simulink model "SS6_Estimation"  (R2014b)
settings: Solver=ode45  StartTime=0.0  StopTime=50.0  RelTol=1e-3
settings Model: Creator=Bismaya  LastModifiedBy=Bismaya

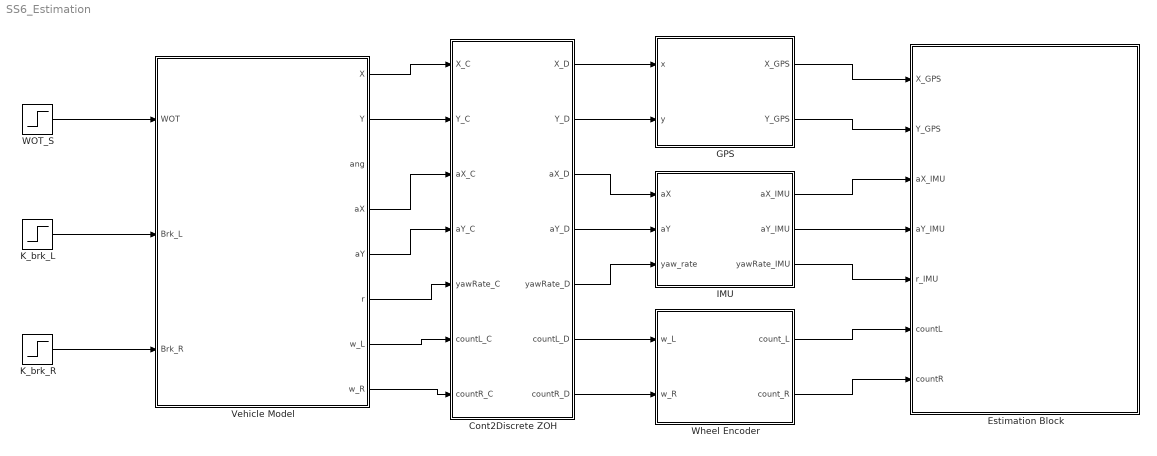
== system SS6_Estimation ==
  Cont2Discrete ZOH : Subsystem
  Estimation Block : Subsystem
  GPS : MATLAB Function  TreatAsAtomicUnit=on
  IMU : MATLAB Function  TreatAsAtomicUnit=on
  K_brk_L : Step  Time=0  After=0  SampleTime=0
  K_brk_R : Step  Time=20  SampleTime=0
  Vehicle Model : Subsystem
  "WOT_S " : Step  Time=0  Before=1  SampleTime=0
  Wheel Encoder : MATLAB Function  TreatAsAtomicUnit=on
  wires:
  "WOT_S "/1 -> Vehicle Model/1(WOT)
  K_brk_L/1 -> Vehicle Model/2(Brk_L)
  K_brk_R/1 -> Vehicle Model/3(Brk_R)
  Vehicle Model/1(X) -> Cont2Discrete ZOH/1(X_C)
  Vehicle Model/2(Y) -> Cont2Discrete ZOH/2(Y_C)
  Vehicle Model/4(aX) -> Cont2Discrete ZOH/3(aX_C)
  Vehicle Model/5(aY) -> Cont2Discrete ZOH/4(aY_C)
  Vehicle Model/6(r) -> Cont2Discrete ZOH/5(yawRate_C)
  Vehicle Model/7(w_L) -> Cont2Discrete ZOH/6(countL_C)
  Cont2Discrete ZOH/1(X_D) -> GPS/1(x)
  Cont2Discrete ZOH/2(Y_D) -> GPS/2(y)
  Cont2Discrete ZOH/3(aX_D) -> IMU/1(aX)
  Cont2Discrete ZOH/4(aY_D) -> IMU/2(aY)
  Cont2Discrete ZOH/5(yawRate_D) -> IMU/3(yaw_rate)
  Cont2Discrete ZOH/6(countL_D) -> Wheel Encoder/1(w_L)
  Cont2Discrete ZOH/7(countR_D) -> Wheel Encoder/2(w_R)
  GPS/1(X_GPS) -> Estimation Block/1(X_GPS)
  GPS/2(Y_GPS) -> Estimation Block/2(Y_GPS)
  IMU/1(aX_IMU) -> Estimation Block/3(aX_IMU)
  IMU/2(aY_IMU) -> Estimation Block/4(aY_IMU)
  IMU/3(yawRate_IMU) -> Estimation Block/5(r_IMU)
  Wheel Encoder/1(count_L) -> Estimation Block/6(countL)
  Wheel Encoder/2(count_R) -> Estimation Block/7(countR)
  Vehicle Model/8(w_R) -> Cont2Discrete ZOH/7(countR_C)

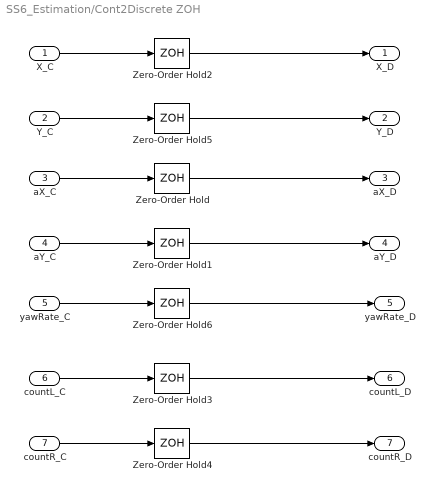
== system SS6_Estimation/Cont2Discrete ZOH ==
  X_C : Inport
  Y_C : Inport  Port=2
  aX_C : Inport  Port=3
  aY_C : Inport  Port=4
  yawRate_C : Inport  Port=5
  countL_C : Inport  Port=6
  countR_C : Inport  Port=7
  Zero-Order Hold{,1..6} (7 alike) : ZeroOrderHold  SampleTime=0.01
  X_D : Outport
  Y_D : Outport  Port=2
  aX_D : Outport  Port=3
  aY_D : Outport  Port=4
  yawRate_D : Outport  Port=5
  countL_D : Outport  Port=6
  countR_D : Outport  Port=7
  wires:
  Zero-Order Hold5/1 -> Y_D/1
  Zero-Order Hold2/1 -> X_D/1
  yawRate_C/1 -> Zero-Order Hold6/1
  aX_C/1 -> Zero-Order Hold/1
  aY_C/1 -> Zero-Order Hold1/1
  Y_C/1 -> Zero-Order Hold5/1
  X_C/1 -> Zero-Order Hold2/1
  countR_C/1 -> Zero-Order Hold4/1
  countL_C/1 -> Zero-Order Hold3/1
  Zero-Order Hold/1 -> aX_D/1
  Zero-Order Hold4/1 -> countR_D/1
  Zero-Order Hold3/1 -> countL_D/1
  Zero-Order Hold6/1 -> yawRate_D/1
  Zero-Order Hold1/1 -> aY_D/1

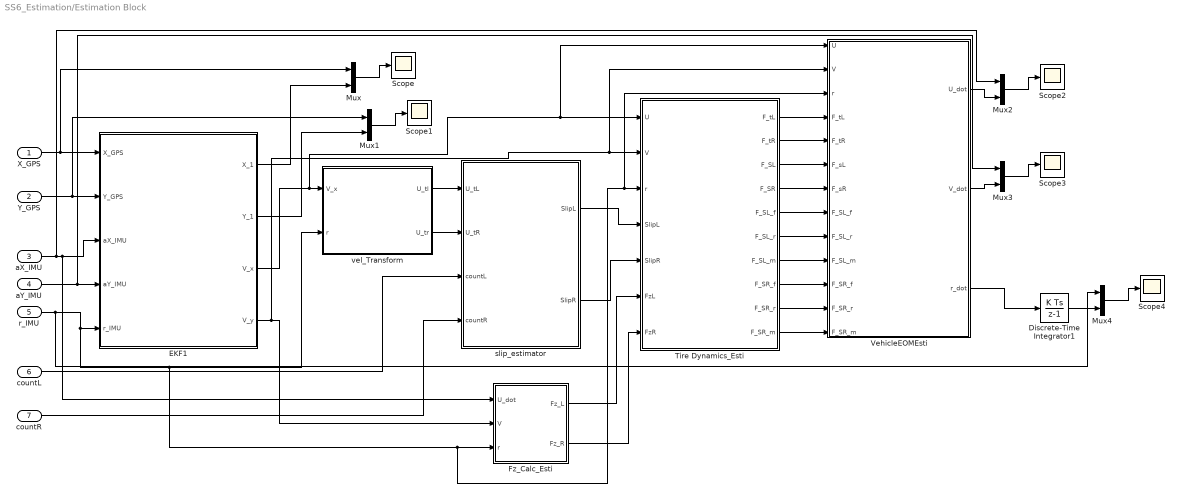
== system SS6_Estimation/Estimation Block ==
  X_GPS : Inport
  Y_GPS : Inport  Port=2
  aX_IMU : Inport  Port=3
  aY_IMU : Inport  Port=4
  r_IMU : Inport  Port=5
  countL : Inport  Port=6
  countR : Inport  Port=7
  Discrete-Time Integrator1 : DiscreteIntegrator  InitialConditionSetting=State (most efficient)  SampleTime=-1
  EKF1 : MATLAB Function  TreatAsAtomicUnit=on
  Fz_Calc_Esti : MATLAB Function  TreatAsAtomicUnit=on
  Mux{,1..4} (5 alike) : Mux  Inputs=2
  Scope{,1..4} (5 alike) : Scope
      Scope settings: SaveName=X_Comp
      Scope1 settings: SaveName=YComp
      Scope2 settings: SaveName=X_Comp1
      Scope3 settings: SaveName=X_Comp2
      Scope4 settings: SaveName=X_Comp3
  Tire Dynamics_Esti : Subsystem
  VehicleEOMEsti : MATLAB Function  TreatAsAtomicUnit=on
  slip_estimator : MATLAB Function  TreatAsAtomicUnit=on
  vel_Transform : MATLAB Function  TreatAsAtomicUnit=on
  wires:
  slip_estimator/1(SlipL) -> Tire Dynamics_Esti/4(SlipL)
  Tire Dynamics_Esti/10(F_SR_m) -> VehicleEOMEsti/13(F_SR_m)
  slip_estimator/2(SlipR) -> Tire Dynamics_Esti/5(SlipR)
  X_GPS/1 -> Mux/1, EKF1/1(X_GPS)
  aY_IMU/1 -> Mux3/1, EKF1/4(aY_IMU)
  aX_IMU/1 -> Mux2/1, Fz_Calc_Esti/1(U_dot), EKF1/3(aX_IMU)
  vel_Transform/2(U_tr) -> slip_estimator/2(U_tR)
  vel_Transform/1(U_tl) -> slip_estimator/1(U_tL)
  Fz_Calc_Esti/2(Fz_R) -> Tire Dynamics_Esti/7(FzR)
  Tire Dynamics_Esti/7(F_SL_m) -> VehicleEOMEsti/10(F_SL_m)
  Tire Dynamics_Esti/6(F_SL_r) -> VehicleEOMEsti/9(F_SL_r)
  Tire Dynamics_Esti/9(F_SR_r) -> VehicleEOMEsti/12(F_SR_r)
  Tire Dynamics_Esti/8(F_SR_f) -> VehicleEOMEsti/11(F_SR_f)
  Tire Dynamics_Esti/5(F_SL_f) -> VehicleEOMEsti/8(F_SL_f)
  Fz_Calc_Esti/1(Fz_L) -> Tire Dynamics_Esti/6(FzL)
  Tire Dynamics_Esti/1(F_tL) -> VehicleEOMEsti/4(F_tL)
  Tire Dynamics_Esti/3(F_SL) -> VehicleEOMEsti/6(F_sL)
  Tire Dynamics_Esti/2(F_tR) -> VehicleEOMEsti/5(F_tR)
  Tire Dynamics_Esti/4(F_SR) -> VehicleEOMEsti/7(F_sR)
  Mux/1 -> Scope/1
  EKF1/1(X_1) -> Mux/2
  Y_GPS/1 -> Mux1/1, EKF1/2(Y_GPS)
  Mux1/1 -> Scope1/1
  EKF1/2(Y_1) -> Mux1/2
  countL/1 -> slip_estimator/3(countL)
  countR/1 -> slip_estimator/4(countR)
  EKF1/3(V_x) -> VehicleEOMEsti/1(U), Tire Dynamics_Esti/1(U), vel_Transform/1(V_x)
  EKF1/4(V_y) -> VehicleEOMEsti/2(V), Tire Dynamics_Esti/2(V), Fz_Calc_Esti/2(V)
  r_IMU/1 -> Mux4/1, VehicleEOMEsti/3(r), Tire Dynamics_Esti/3(r), Fz_Calc_Esti/3(r), vel_Transform/2(r), EKF1/5(r_IMU)
  Mux2/1 -> Scope2/1
  VehicleEOMEsti/1(U_dot) -> Mux2/2
  Mux3/1 -> Scope3/1
  VehicleEOMEsti/2(V_dot) -> Mux3/2
  Mux4/1 -> Scope4/1
  Discrete-Time Integrator1/1 -> Mux4/2
  VehicleEOMEsti/3(r_dot) -> Discrete-Time Integrator1/1

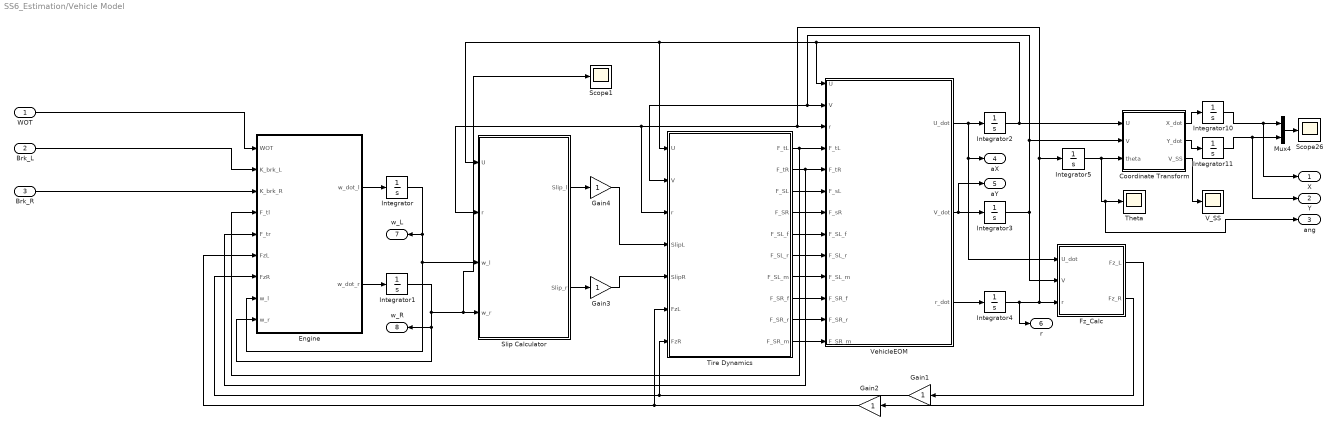
== system SS6_Estimation/Vehicle Model ==
  WOT : Inport
  Brk_L : Inport  Port=2
  Brk_R : Inport  Port=3
  Coordinate Transform : MATLAB Function  TreatAsAtomicUnit=on
  Engine : MATLAB Function  TreatAsAtomicUnit=on
  Fz_Calc : MATLAB Function  TreatAsAtomicUnit=on
  Gain{1..4} (4 alike) : Gain
  Integrator : Integrator  InitialCondition=12  LowerSaturationLimit=-0.0001
  Integrator1 : Integrator  InitialCondition=12  LowerSaturationLimit=-0.0001
  Integrator{3..5,10..11} (5 alike) : Integrator
  Integrator2 : Integrator  InitialCondition=10/3
  Mux4 : Mux  Inputs=2
  Scope1 : Scope
      settings: YMin=-50  YMax=200  SaveName=XY1
  Scope26 : Scope
      settings: YMin=-50  YMax=200  SaveName=XY
  Slip Calculator : MATLAB Function  TreatAsAtomicUnit=on
  Theta : Scope
      settings: YMin=20  YMax=45  SaveName=Theta
  Tire Dynamics : Subsystem
  V_SS : Scope
      settings: YMin=20  YMax=45  SaveName=Theta1
  VehicleEOM : MATLAB Function  TreatAsAtomicUnit=on
  X : Outport
  Y : Outport  Port=2
  ang : Outport  Port=3
  aX : Outport  Port=4
  aY : Outport  Port=5
  r : Outport  Port=6
  w_L : Outport  Port=7
  w_R : Outport  Port=8
  wires:
  Engine/1(w_dot_l) -> Integrator/1
  Integrator1/1 -> w_R/1, Engine/9(w_r), Scope1/1, Slip Calculator/4(w_r)
  Tire Dynamics/9(F_SR_r) -> VehicleEOM/12(F_SR_r)
  Tire Dynamics/8(F_SR_f) -> VehicleEOM/11(F_SR_f)
  Tire Dynamics/5(F_SL_f) -> VehicleEOM/8(F_SL_f)
  Tire Dynamics/7(F_SL_m) -> VehicleEOM/10(F_SL_m)
  Brk_L/1 -> Engine/2(K_brk_L)
  Integrator/1 -> w_L/1, Slip Calculator/3(w_l), Engine/8(w_l)
  Brk_R/1 -> Engine/3(K_brk_R)
  Tire Dynamics/1(F_tL) -> Engine/4(F_tl), VehicleEOM/4(F_tL)
  Engine/2(w_dot_r) -> Integrator1/1
  Tire Dynamics/4(F_SR) -> VehicleEOM/7(F_sR)
  VehicleEOM/1(U_dot) -> aX/1, Fz_Calc/1(U_dot), Integrator2/1
  VehicleEOM/2(V_dot) -> aY/1, Integrator3/1
  VehicleEOM/3(r_dot) -> Integrator4/1
  Integrator2/1 -> Tire Dynamics/1(U), Slip Calculator/1(U), VehicleEOM/1(U), Coordinate Transform/1(U)
  Integrator3/1 -> Tire Dynamics/2(V), VehicleEOM/2(V), Coordinate Transform/2(V), Fz_Calc/2(V)
  Fz_Calc/2(Fz_R) -> Gain1/1
  Fz_Calc/1(Fz_L) -> Gain2/1
  Slip Calculator/2(Slip_r) -> Gain3/1
  Tire Dynamics/2(F_tR) -> Engine/5(F_tr), VehicleEOM/5(F_tR)
  Integrator4/1 -> r/1, Tire Dynamics/3(r), Slip Calculator/2(r), VehicleEOM/3(r), Integrator5/1, Fz_Calc/3(r)
  Integrator5/1 -> Coordinate Transform/3(theta), ang/1, Theta/1
  Coordinate Transform/1(X_dot) -> Integrator10/1
  Slip Calculator/1(Slip_l) -> Gain4/1
  WOT/1 -> Engine/1(WOT)
  Tire Dynamics/10(F_SR_m) -> VehicleEOM/13(F_SR_m)
  Tire Dynamics/6(F_SL_r) -> VehicleEOM/9(F_SL_r)
  Tire Dynamics/3(F_SL) -> VehicleEOM/6(F_sL)
  Gain1/1 -> Engine/7(FzR), Tire Dynamics/7(FzR)
  Gain3/1 -> Tire Dynamics/5(SlipR)
  Gain2/1 -> Engine/6(FzL), Tire Dynamics/6(FzL)
  Gain4/1 -> Tire Dynamics/4(SlipL)
  Coordinate Transform/2(Y_dot) -> Integrator11/1
  Integrator10/1 -> X/1, Mux4/1
  Integrator11/1 -> Y/1, Mux4/2
  Mux4/1 -> Scope26/1
  Coordinate Transform/3(V_SS) -> V_SS/1

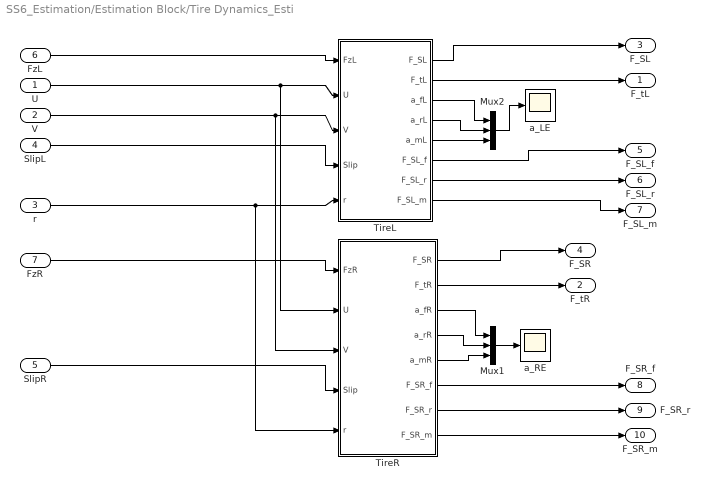
== system SS6_Estimation/Estimation Block/Tire Dynamics_Esti ==
  U : Inport
  V : Inport  Port=2
  r : Inport  Port=3
  SlipL : Inport  Port=4
  SlipR : Inport  Port=5
  FzL : Inport  Port=6
  FzR : Inport  Port=7
  Mux1 : Mux  Inputs=3
  Mux2 : Mux  Inputs=3
  TireL : MATLAB Function  TreatAsAtomicUnit=on
  TireR : MATLAB Function  TreatAsAtomicUnit=on
  a_LE : Scope
      settings: YMin=20  YMax=45  SaveName=a_LE  MaxDataPoints=5000000
  a_RE : Scope
      settings: YMin=20  YMax=45  SaveName=a_RE  MaxDataPoints=5000000
  F_tL : Outport
  F_tR : Outport  Port=2
  F_SL : Outport  Port=3
  F_SR : Outport  Port=4
  F_SL_f : Outport  Port=5
  F_SL_r : Outport  Port=6
  F_SL_m : Outport  Port=7
  F_SR_f : Outport  Port=8
  F_SR_r : Outport  Port=9
  F_SR_m : Outport  Port=10
  wires:
  TireL/8(F_SL_m) -> F_SL_m/1
  U/1 -> TireL/2(U), TireR/2(U)
  FzR/1 -> TireR/1(FzR)
  SlipR/1 -> TireR/4(Slip)
  V/1 -> TireR/3(V), TireL/3(V)
  TireR/1(F_SR) -> F_SR/1
  r/1 -> TireR/5(r), TireL/5(r)
  TireL/2(F_tL) -> F_tL/1
  TireL/6(F_SL_f) -> F_SL_f/1
  SlipL/1 -> TireL/4(Slip)
  TireL/7(F_SL_r) -> F_SL_r/1
  FzL/1 -> TireL/1(FzL)
  TireL/1(F_SL) -> F_SL/1
  Mux2/1 -> a_LE/1
  TireR/3(a_fR) -> Mux1/1
  TireR/4(a_rR) -> Mux1/2
  Mux1/1 -> a_RE/1
  TireR/5(a_mR) -> Mux1/3
  TireR/2(F_tR) -> F_tR/1
  TireR/6(F_SR_f) -> F_SR_f/1
  TireR/7(F_SR_r) -> F_SR_r/1
  TireR/8(F_SR_m) -> F_SR_m/1
  TireL/5(a_mL) -> Mux2/3
  TireL/3(a_fL) -> Mux2/1
  TireL/4(a_rL) -> Mux2/2

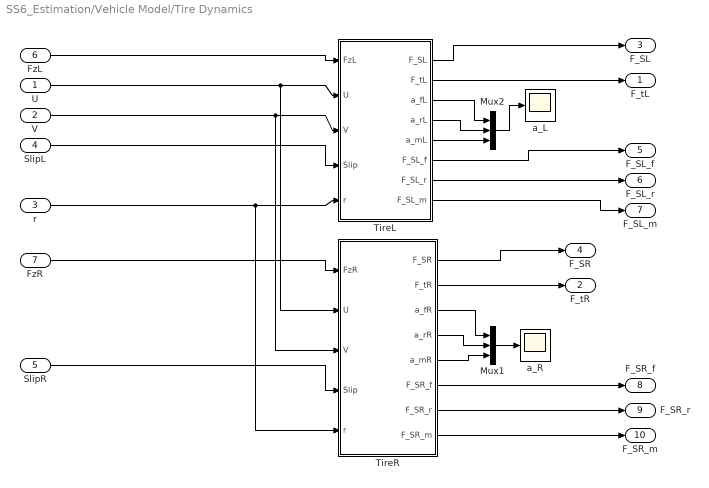
== system SS6_Estimation/Vehicle Model/Tire Dynamics ==
  U : Inport
  V : Inport  Port=2
  r : Inport  Port=3
  SlipL : Inport  Port=4
  SlipR : Inport  Port=5
  FzL : Inport  Port=6
  FzR : Inport  Port=7
  Mux1 : Mux  Inputs=3
  Mux2 : Mux  Inputs=3
  TireL : MATLAB Function  TreatAsAtomicUnit=on
  TireR : MATLAB Function  TreatAsAtomicUnit=on
  a_L : Scope
      settings: YMin=20  YMax=45  SaveName=a_L  MaxDataPoints=5000000
  a_R : Scope
      settings: YMin=20  YMax=45  SaveName=a_R  MaxDataPoints=5000000
  F_tL : Outport
  F_tR : Outport  Port=2
  F_SL : Outport  Port=3
  F_SR : Outport  Port=4
  F_SL_f : Outport  Port=5
  F_SL_r : Outport  Port=6
  F_SL_m : Outport  Port=7
  F_SR_f : Outport  Port=8
  F_SR_r : Outport  Port=9
  F_SR_m : Outport  Port=10
  wires:
  TireL/8(F_SL_m) -> F_SL_m/1
  U/1 -> TireL/2(U), TireR/2(U)
  FzR/1 -> TireR/1(FzR)
  SlipR/1 -> TireR/4(Slip)
  V/1 -> TireR/3(V), TireL/3(V)
  TireR/1(F_SR) -> F_SR/1
  r/1 -> TireR/5(r), TireL/5(r)
  TireL/2(F_tL) -> F_tL/1
  TireL/6(F_SL_f) -> F_SL_f/1
  SlipL/1 -> TireL/4(Slip)
  TireL/7(F_SL_r) -> F_SL_r/1
  FzL/1 -> TireL/1(FzL)
  TireL/1(F_SL) -> F_SL/1
  Mux2/1 -> a_L/1
  TireR/3(a_fR) -> Mux1/1
  TireR/4(a_rR) -> Mux1/2
  Mux1/1 -> a_R/1
  TireR/5(a_mR) -> Mux1/3
  TireR/2(F_tR) -> F_tR/1
  TireR/6(F_SR_f) -> F_SR_f/1
  TireR/7(F_SR_r) -> F_SR_r/1
  TireR/8(F_SR_m) -> F_SR_m/1
  TireL/5(a_mL) -> Mux2/3
  TireL/3(a_fL) -> Mux2/1
  TireL/4(a_rL) -> Mux2/2

== matlab function SS6_Estimation/GPS ==
  data: x input; y input; X_GPS output; Y_GPS output
function [X_GPS,Y_GPS] = GPS_fcn(x,y)
%#codegen

X_GPS=x+0.0001*randn(1);
Y_GPS=y+0.0001*randn(1);

== matlab function SS6_Estimation/Vehicle Model/Engine ==
  data: WOT input; K_brk_L input; K_brk_R input; F_tl input; F_tr input; FzL input; FzR input; w_l input; w_r input; w_dot_l output; w_dot_r output
function [w_dot_l,w_dot_r] = engine_model(WOT,K_brk_L,K_brk_R,F_tl,F_tr,FzL,FzR,w_l,w_r)
M=1280;Ms=1160;Izz=2500;Ixx=750;Ixz=0;a=1.203;b=1.217;hcg=0.5;e=0.2;Tw=1.33;R=0.3;I_t=2.1;
I_e=0.136;A_f=2.1;zi1=2.5*13.56;zi2=7.50;zi3=5.37;zi4=4.22;zi5=3.28;
Lbpsi=45000;Lbp=2600;C_a=20000;C_i=20000;mu=0.85;e_r=0.015;K_rsf=-0.05;K_rsr=0.1;
C1=-6.0;C2=59.16;C3=25;C_s1=1.38;K_rsf=0.444;C_d=0.32;d=0.014;n=0.85;
rho=1.204;g=9.81;
K_bf=0.55;
zi=zi1*2;

F_tl=F_tl;
F_tr=F_tr;
F_t1=F_tl+F_tr;
%Engine Equations
w_el=zi*w_l;
w_er=zi*w_r;

IwL=I_t+(0.5*zi*zi*n*I_e);%Accelerating
IwR=I_t+(0.5*zi*zi*n*I_e);%Accelerating

T_l=WOT*zi*n*(C1*(w_el/100)^2+C2*(w_el/100)+C3);
T_r=WOT*zi*n*(C1*(w_er/100)^2+C2*(w_er/100)+C3);
T_trac_L=T_l-(R*F_tl)-(d*FzL);
T_trac_R=T_r-(R*F_tr)-(d*FzR);
T_brkl=K_brk_L*T_l;
T_brkr=K_brk_R*T_r;
w_dot_l=(1/(IwL))*(T_trac_L-T_brkl);
w_dot_r=(1/(IwR))*(T_trac_R-T_brkr);
% w_dot_f=(1/Iw)*(T_f-(d*Fzf)-(0.5*T_brkf));
% w_dot_r=(1/Iw)*(T_r-(d*Fzr)-(0.5*T_brkr));

== matlab function SS6_Estimation/Vehicle Model/Tire Dynamics/TireR ==
  data: FzR input; F_SR output; F_tR output; U input; V input; Slip input; r input; a_fR output; a_rR output; a_mR output; F_SR_f output; F_SR_r output; F_SR_m output
function [F_SR,F_tR,a_fR,a_rR,a_mR,F_SR_f,F_SR_r,F_SR_m] = tireR(FzR,U,V,Slip,r)
M=1280;Ms=1160;Izz=2500;Ixx=750;Ixz=0;a=1.203;b=1.217;hcg=0.5;e=0.2;Tw=1.33;R=0.3;I_t=2.1;
I_e=0.136;A_f=2.1;K_bf=0.55;zi1=13.56;z2=7.50;zi3=5.37;zi4=4.22;zi5=3.28;
Lbpsi=45000;Lbp=2600;C_a=20000;C_i=20000;mu=0.85;e_r=0.015;K_rsf=-0.05;K_rsr=0.1;
C1=-6.0;C2=59.16;C3=25;C_s1=1.38;K_rsf=0.444;C_d=0.32;d=0.014;n=0.85;
rho=1.204;g=9.81;c=0.2;


% FzF=M*g*mu/2;
Fz=FzR;

%Tire Longitudinal Velocity Calculation
% U_tf=U*cos(delta)+(V+a*r)*sin(delta);
% U_tr=U;

 %Side Slip Calc
a_fR=-atan((V+a*r)/(U-0.5*Tw*r));
a_rR=atan((b*r-V)/(U-0.5*Tw*r));
a_mR=atan((c*r-V)/(U-0.5*Tw*r));

alpha=a_fR;

 U_tl=U+(0.5*Tw*r);
 U_tr=U-(0.5*Tw*r);
%%FRONT Tires
%Tire Equations
S_f=(mu*(Fz/3)*(1-(e_r*U_tr*sqrt((Slip*Slip)+(tan(alpha)*tan(alpha)))))*(1-Slip))/...
    (2*sqrt(C_i*C_i*Slip*Slip+C_a*C_a*tan(alpha)*tan(alpha)));
if(S_f<1)
    f_S=S_f*(2-S_f);
else
    f_S=1;
end
F_SR_f=(C_a*tan(alpha)*f_S)/(1-Slip);
F_tR_f=(C_i*Slip*f_S)/(1-Slip);

%%Rear Tires
alpha=a_rR;

S_r=(mu*(Fz/3)*(1-(e_r*U_tr*sqrt((Slip*Slip)+(tan(alpha)*tan(alpha)))))*(1-Slip))/...
    (2*sqrt(C_i*C_i*Slip*Slip+C_a*C_a*tan(alpha)*tan(alpha)));
if(S_r<1)
    f_S=S_r*(2-S_r);
else
    f_S=1;
end
F_SR_r=(C_a*tan(alpha)*f_S)/(1-Slip);
F_tR_r=(C_i*Slip*f_S)/(1-Slip);

%%Middle Tires
alpha=a_mR;

S_m=(mu*(Fz/3)*(1-(e_r*U_tr*sqrt((Slip*Slip)+(tan(alpha)*tan(alpha)))))*(1-Slip))/...
    (2*sqrt(C_i*C_i*Slip*Slip+C_a*C_a*tan(alpha)*tan(alpha)));
if(S_m<1)
    f_S=S_m*(2-S_m);
else
    f_S=1;
end
F_SR_m=(C_a*tan(alpha)*f_S)/(1-Slip);
F_tR_m=(C_i*Slip*f_S)/(1-Slip);


F_SR=F_SR_f+F_SR_r+F_SR_m;
F_tR=F_tR_f+F_tR_r+F_tR_m;
F_R=[F_tR_f;F_tR_r;F_tR_m;F_SR_f;F_SR_r;F_SR_m];

== matlab function SS6_Estimation/Vehicle Model/VehicleEOM ==
  data: U input; V input; U_dot output; V_dot output; r input; F_tL input; F_tR input; F_sL input; F_sR input; r_dot output; F_SL_f input; F_SL_r input; F_SL_m input; F_SR_f input; F_SR_r input; F_SR_m input
function [U_dot,V_dot,r_dot] = VehicleEOM(U,V,r,F_tL,F_tR,F_sL,F_sR,F_SL_f,F_SL_r,F_SL_m,F_SR_f,F_SR_r,F_SR_m)
M=1280;Ms=1160;Izz=2500;Ixx=750;Ixz=0;a=1.203;b=1.217;hcg=0.5;e=0.2;Tw=1.33;R=0.3;I_t=2.1;
I_e=0.136;A_f=2.1;K_bf=0.55;zi1=13.56;z2=7.50;zi3=5.37;zi4=4.22;zi5=3.28;
Lbpsi=45000;Lbp=2600;C_a=20000;C_i=20000;mu=0.85;e_r=0.015;K_rsf=-0.05;K_rsr=0.1;
C1=-6.0;C2=59.16;C3=25;C_s1=1.38;K_rsf=0.444;C_d=0.32;d=0.014;n=0.85;
rho=1.204;g=9.81;c=0.2;

F_t=(F_tL+F_tR);
%Vehicle Equations
% U_dot=(1/M)*((M*V*r)+F_t-(0.5*C_d*A_f*rho*U*U));
U_dot=(1/M)*((M*V*r)+F_t);

V_dot=(1/M)*((-M*U*r)+F_sL+F_sR);
% r_dot=(1/Izz)*(2*a*F_tL*sin(delta)+2*a*F_sL*cos(delta)-2*b*F_sR);
 r_dot=(1/(0.5*Izz))*(0.5*Tw*F_tL-0.5*Tw*F_tR+a*(F_SL_f+F_SR_f)-b*(F_SL_r+F_SR_r)-c*(F_SL_m+F_SR_m));

== matlab function SS6_Estimation/Vehicle Model/Slip Calculator ==
  data: U input; r input; w_l input; w_r input; Slip_l output; Slip_r output
function [Slip_l,Slip_r] = slipCalculator(U,r,w_l,w_r)
M=1280;Ms=1160;Izz=2500;Ixx=750;Ixz=0;a=1.203;b=1.217;hcg=0.5;e=0.2;Tw=1.33;R=0.3;I_t=2.1;
I_e=0.136;A_f=2.1;K_bf=0.55;zi1=13.56;z2=7.50;zi3=5.37;zi4=4.22;zi5=3.28;
Lbpsi=45000;Lbp=2600;C_a=20000;C_i=20000;mu=0.85;e_r=0.015;K_rsf=-0.05;K_rsr=0.1;
C1=-6.0;C2=59.16;C3=25;C_s1=1.38;K_rsf=0.444;C_d=0.32;d=0.014;n=0.85;
rho=1.204;g=9.81;

% w_r=-w_r;
% w_f=-w_f;
%Tire Longitudinal Velocity Calculation
% U_tl=U*cos(delta)+(V+a*r)*sin(delta);
% U_tr=U;
 U_tl=U+(0.5*Tw*r);
 U_tr=U-(0.5*Tw*r);

% %  SlipCalc
% if(U_tl<=(R*w_l))
%     Slip_l=1-(U_tl/(R*w_l));%Acceleration
% else
%     Slip_l=1-((R*w_l)/U_tl);%Braking
% %     Slip_l=0;
% end
% 
% if(U_tr<=(R*w_r))
%     Slip_r=1-(U_tr/(R*w_r));%Acceleration
% else
%     Slip_r=1-((R*w_r)/U_tr);%Braking
% %     Slip_r=0;
% end
Slip_l=1-(U_tl/(R*w_l));
Slip_r=1-(U_tr/(R*w_r));

% 
% if(Slip_l<0)
%      Slip_l=0;
%  elseif (Slip_l>1)
%          Slip_l=1;
%  end
%  if(Slip_r<0)
%      Slip_r=0;
%  elseif (Slip_r>1)
%          Slip_r=1;
%  end
% %

== matlab function SS6_Estimation/Vehicle Model/Fz_Calc ==
  data: U_dot input; V input; Fz_L output; Fz_R output; r input
function [Fz_L,Fz_R] = FzCalc(U_dot,V,r)
M=1280;Ms=1160;Izz=2500;Ixx=750;Ixz=0;a=1.203;b=1.217;hcg=0.5;e=0.2;Tw=1.33;R=0.3;I_t=2.1;
I_e=0.136;A_f=2.1;K_bf=0.55;zi1=13.56;z2=7.50;zi3=5.37;zi4=4.22;zi5=3.28;
Lbpsi=45000;Lbp=2600;C_a=20000;C_i=20000;mu=0.85;e_r=0.015;K_rsf=-0.05;K_rsr=0.1;
C1=-6.0;C2=59.16;C3=25;C_s1=1.38;K_rsf=0.444;C_d=0.32;d=0.014;n=0.85;
rho=1.204;g=9.81;


%NormalForceCalc
% Fz_f=(M*g/2)*((b/(a+b))-((U_dot-V*r)*hcg)/(g*(a+b)));
% Fz_r=(M*g/2)*((a/(a+b))+((U_dot-V*r)*hcg)/(g*(a+b)));
Fz_L=(M*g/2);
Fz_R=(M*g/2);

== matlab function SS6_Estimation/Vehicle Model/Tire Dynamics/TireL ==
  data: FzL input; F_SL output; F_tL output; U input; V input; Slip input; r input; a_fL output; a_rL output; a_mL output; F_SL_f output; F_SL_r output; F_SL_m output
function [F_SL,F_tL,a_fL,a_rL,a_mL,F_SL_f,F_SL_r,F_SL_m] = tireL(FzL,U,V,Slip,r)
M=1280;Ms=1160;Izz=2500;Ixx=750;Ixz=0;a=1.203;b=1.217;hcg=0.5;e=0.2;Tw=1.33;R=0.3;I_t=2.1;
I_e=0.136;A_f=2.1;K_bf=0.55;zi1=13.56;z2=7.50;zi3=5.37;zi4=4.22;zi5=3.28;
Lbpsi=45000;Lbp=2600;C_a=20000;C_i=20000;mu=0.85;e_r=0.015;K_rsf=-0.05;K_rsr=0.1;
C1=-6.0;C2=59.16;C3=25;C_s1=1.38;K_rsf=0.444;C_d=0.32;d=0.014;n=0.85;
rho=1.204;g=9.81;c=0.2;


% FzF=M*g*mu/2;

Fz=FzL;

%Tire Longitudinal Velocity Calculation
% U_tf=U*cos(delta)+(V+a*r)*sin(delta);
% U_tr=U;
 U_tl=U+(0.5*Tw*r);
 U_tr=U-(0.5*Tw*r);
%FRONT Tires
 %Side Slip Calc
a_fL=-atan((V+a*r)/(U+0.5*Tw*r));
a_rL=atan((b*r-V)/(U+0.5*Tw*r));
a_mL=atan((c*r-V)/(U+0.5*Tw*r));

alpha=a_fL;
%Tire Equations
S_f=(mu*(Fz/3)*(1-(e_r*U_tl*sqrt((Slip*Slip)+(tan(alpha)*tan(alpha)))))*(1-Slip))/...
    (2*sqrt(C_i*C_i*Slip*Slip+C_a*C_a*tan(alpha)*tan(alpha)));
if(S_f<1)
    f_S=S_f*(2-S_f);
else
    f_S=1;
end
F_SL_f=(C_a*tan(alpha)*f_S)/(1-Slip);
F_tL_f=(C_i*Slip*f_S)/(1-Slip);

%Rear Tires
alpha=a_rL;

S_r=(mu*(Fz/3)*(1-(e_r*U_tl*sqrt((Slip*Slip)+(tan(alpha)*tan(alpha)))))*(1-Slip))/...
    (2*sqrt(C_i*C_i*Slip*Slip+C_a*C_a*tan(alpha)*tan(alpha)));
if(S_r<1)
    f_S=S_r*(2-S_r);
else
    f_S=1;
end
F_SL_r=(C_a*tan(alpha)*f_S)/(1-Slip);
F_tL_r=(C_i*Slip*f_S)/(1-Slip);

%Middle Tires
alpha=a_mL;

S_m=(mu*(Fz/3)*(1-(e_r*U_tl*sqrt((Slip*Slip)+(tan(alpha)*tan(alpha)))))*(1-Slip))/...
    (2*sqrt(C_i*C_i*Slip*Slip+C_a*C_a*tan(alpha)*tan(alpha)));
if(S_m<1)
    f_S=S_m*(2-S_m);
else
    f_S=1;
end
F_SL_m=(C_a*tan(alpha)*f_S)/(1-Slip);
F_tL_m=(C_i*Slip*f_S)/(1-Slip);


F_SL=F_SL_f+F_SL_r+F_SL_m;
F_tL=F_tL_f+F_tL_r+F_tL_m;
F_L=[F_tL_f;F_tL_r;F_tL_m;F_SL_f;F_SL_r;F_SL_m;];

== matlab function SS6_Estimation/Vehicle Model/Coordinate Transform ==
  data: U input; V input; theta input; X_dot output; Y_dot output; V_SS output
    function [X_dot,Y_dot, V_SS] = CT(U,V,theta)
M=1280;Ms=1160;Izz=2500;Ixx=750;Ixz=0;a=1.203;b=1.217;hcg=0.5;e=0.2;Tw=1.33;R=0.3;I_t=2.1;
I_e=0.136;A_f=2.1;K_bf=0.55;zi1=13.56;z2=7.50;zi3=5.37;zi4=4.22;zi5=3.28;
Lbpsi=45000;Lbp=2600;C_a=20000;C_i=20000;mu=0.85;e_r=0.015;K_rsf=-0.05;K_rsr=0.1;
C1=-6.0;C2=59.16;C3=25;C_s1=1.38;K_rsf=0.444;C_d=0.32;d=0.014;n=0.85;
rho=1.204;g=9.81;c=0.2;

X_dot=U*cos(theta)-V*sin(theta);
Y_dot=+U*sin(theta)+V*cos(theta);
% X_dot=U*sin(theta)+V*cos(theta);
% Y_dot=U*cos(theta)-V*sin(theta);
V_SS=atand(V/U);

== matlab function SS6_Estimation/IMU ==
  data: aX input; aY input; aX_IMU output; aY_IMU output; yaw_rate input; yawRate_IMU output
function [aX_IMU,aY_IMU,yawRate_IMU] = IMU_fcn(aX,aY,yaw_rate)
%#codegen

aX_IMU=aX+0.0001*randn(1);
aY_IMU=aY+0.0001*randn(1);
yawRate_IMU=yaw_rate+0.0001*randn(1);

== matlab function SS6_Estimation/Wheel Encoder ==
  data: w_L input; w_R input; count_L output; count_R output
function [count_L,count_R] = encoder_fcn(w_L,w_R)
%#codegen

count_L=w_L+0.0001*randn(1);
count_R=w_R+0.0001*randn(1);

== matlab function SS6_Estimation/Estimation Block/EKF1 ==
  data: X_1 output; Y_1 output; X_GPS input; Y_GPS input; aX_IMU input; aY_IMU input; r_IMU input; V_x output; V_y output
function [X_1,Y_1,V_x,V_y]  = EKF_fcn(X_GPS,Y_GPS,aX_IMU,aY_IMU,r_IMU)

persistent cov State 

if isempty(cov)
State=zeros(7,1);
cov=zeros(7);
end

% Motion Noise
Q=0.0001*eye(7);
Q(4:7,4:7)=0;
% Measurement Noise
R=0.0001*eye(2);
% Sampling Time
Ts=0.01;
% Control Matrix
B=[Ts 0 0;
    0 Ts 0;
    0 0 Ts;
    0 0 0;
    0 0 0;
    0 0 0;
    0 0 0;];

%Motion Jacobian
G=[ 1 0 0 0 0 0 0;
    0 1 0 0 0 0 0;
    0 0 1 0 0 0 0;
    cos(State(3)) -sin(State(3)) -State(1)*sin(State(3))-State(2)*cos(State(3)) 0 0 0 0;
    sin(State(3)) cos(State(3)) State(1)*cos(State(3))-State(2)*sin(State(3)) 0 0 0 0;
    0 0 0 Ts 0 1 0;
    0 0 0 0 Ts 0 1;];

% Motion Model 
g=[State(1);
    State(2);
    State(3);
    State(1)*cos(State(3))-State(2)*sin(State(3));
    State(1)*sin(State(3))+State(2)*cos(State(3));
    Ts*State(4)+State(6);
    Ts*State(5)+State(7);];

%Propagate the State and Covariance
State_p=g+B*[aX_IMU;
             aY_IMU;
             r_IMU;];
cov=G*cov*G'+Q;

H= [0 0 0 0 0 1 0;
    0 0 0 0 0 0 1;];
%     0 0 1 0 0 0 0;];
% Take Measurements
y_meas=[X_GPS;
        Y_GPS];
    
K=cov*H'*pinv(H*cov*H'+R);
State=State_p+K*(y_meas-H*State_p);
cov = (eye(7)-K*H)*cov;
X_1=State(6);
Y_1=State(7);
V_x=State(1);
V_y=State(2);
end

== matlab function SS6_Estimation/Estimation Block/vel_Transform ==
  data: V_x input; r input; U_tl output; U_tr output
function [U_tl,U_tr] = velocity_transform(V_x,r)
%#codegen
 Tw=1.33;
 U_tl=V_x+(0.5*Tw*r);
 U_tr=V_x-(0.5*Tw*r);
end

== matlab function SS6_Estimation/Estimation Block/slip_estimator ==
  data: U_tL input; U_tR input; SlipL output; SlipR output; countL input; countR input
function [SlipL,SlipR] = slip_estimator(U_tL,U_tR,countL,countR)
%#codegen
R=0.3;

SlipL=1-(U_tL/(R*countL));
SlipR=1-(U_tR/(R*countR));
end

== matlab function SS6_Estimation/Estimation Block/Tire Dynamics_Esti/TireL ==
  data: FzL input; F_SL output; F_tL output; U input; V input; Slip input; r input; a_fL output; a_rL output; a_mL output; F_SL_f output; F_SL_r output; F_SL_m output
function [F_SL,F_tL,a_fL,a_rL,a_mL,F_SL_f,F_SL_r,F_SL_m] = tireL(FzL,U,V,Slip,r)
M=1280;Ms=1160;Izz=2500;Ixx=750;Ixz=0;a=1.203;b=1.217;hcg=0.5;e=0.2;Tw=1.33;R=0.3;I_t=2.1;
I_e=0.136;A_f=2.1;K_bf=0.55;zi1=13.56;z2=7.50;zi3=5.37;zi4=4.22;zi5=3.28;
Lbpsi=45000;Lbp=2600;C_a=20000;C_i=20000;mu=0.85;e_r=0.015;K_rsf=-0.05;K_rsr=0.1;
C1=-6.0;C2=59.16;C3=25;C_s1=1.38;K_rsf=0.444;C_d=0.32;d=0.014;n=0.85;
rho=1.204;g=9.81;c=0.2;


% FzF=M*g*mu/2;

Fz=FzL;

%Tire Longitudinal Velocity Calculation
% U_tf=U*cos(delta)+(V+a*r)*sin(delta);
% U_tr=U;
 U_tl=U+(0.5*Tw*r);
 U_tr=U-(0.5*Tw*r);
%FRONT Tires
 %Side Slip Calc
a_fL=-atan((V+a*r)/(U+0.5*Tw*r));
a_rL=atan((b*r-V)/(U+0.5*Tw*r));
a_mL=atan((c*r-V)/(U+0.5*Tw*r));

alpha=a_fL;
%Tire Equations
S_f=(mu*(Fz/3)*(1-(e_r*U_tl*sqrt((Slip*Slip)+(tan(alpha)*tan(alpha)))))*(1-Slip))/...
    (2*sqrt(C_i*C_i*Slip*Slip+C_a*C_a*tan(alpha)*tan(alpha)));
if(S_f<1)
    f_S=S_f*(2-S_f);
else
    f_S=1;
end
F_SL_f=(C_a*tan(alpha)*f_S)/(1-Slip);
F_tL_f=(C_i*Slip*f_S)/(1-Slip);

%Rear Tires
alpha=a_rL;

S_r=(mu*(Fz/3)*(1-(e_r*U_tl*sqrt((Slip*Slip)+(tan(alpha)*tan(alpha)))))*(1-Slip))/...
    (2*sqrt(C_i*C_i*Slip*Slip+C_a*C_a*tan(alpha)*tan(alpha)));
if(S_r<1)
    f_S=S_r*(2-S_r);
else
    f_S=1;
end
F_SL_r=(C_a*tan(alpha)*f_S)/(1-Slip);
F_tL_r=(C_i*Slip*f_S)/(1-Slip);

%Middle Tires
alpha=a_mL;

S_m=(mu*(Fz/3)*(1-(e_r*U_tl*sqrt((Slip*Slip)+(tan(alpha)*tan(alpha)))))*(1-Slip))/...
    (2*sqrt(C_i*C_i*Slip*Slip+C_a*C_a*tan(alpha)*tan(alpha)));
if(S_m<1)
    f_S=S_m*(2-S_m);
else
    f_S=1;
end
F_SL_m=(C_a*tan(alpha)*f_S)/(1-Slip);
F_tL_m=(C_i*Slip*f_S)/(1-Slip);


F_SL=F_SL_f+F_SL_r+F_SL_m;
F_tL=F_tL_f+F_tL_r+F_tL_m;
F_L=[F_tL_f;F_tL_r;F_tL_m;F_SL_f;F_SL_r;F_SL_m;];

== matlab function SS6_Estimation/Estimation Block/Tire Dynamics_Esti/TireR ==
  data: FzR input; F_SR output; F_tR output; U input; V input; Slip input; r input; a_fR output; a_rR output; a_mR output; F_SR_f output; F_SR_r output; F_SR_m output
function [F_SR,F_tR,a_fR,a_rR,a_mR,F_SR_f,F_SR_r,F_SR_m] = tireR(FzR,U,V,Slip,r)
M=1280;Ms=1160;Izz=2500;Ixx=750;Ixz=0;a=1.203;b=1.217;hcg=0.5;e=0.2;Tw=1.33;R=0.3;I_t=2.1;
I_e=0.136;A_f=2.1;K_bf=0.55;zi1=13.56;z2=7.50;zi3=5.37;zi4=4.22;zi5=3.28;
Lbpsi=45000;Lbp=2600;C_a=20000;C_i=20000;mu=0.85;e_r=0.015;K_rsf=-0.05;K_rsr=0.1;
C1=-6.0;C2=59.16;C3=25;C_s1=1.38;K_rsf=0.444;C_d=0.32;d=0.014;n=0.85;
rho=1.204;g=9.81;c=0.2;


% FzF=M*g*mu/2;
Fz=FzR;

%Tire Longitudinal Velocity Calculation
% U_tf=U*cos(delta)+(V+a*r)*sin(delta);
% U_tr=U;

 %Side Slip Calc
a_fR=-atan((V+a*r)/(U-0.5*Tw*r));
a_rR=atan((b*r-V)/(U-0.5*Tw*r));
a_mR=atan((c*r-V)/(U-0.5*Tw*r));

alpha=a_fR;

 U_tl=U+(0.5*Tw*r);
 U_tr=U-(0.5*Tw*r);
%%FRONT Tires
%Tire Equations
S_f=(mu*(Fz/3)*(1-(e_r*U_tr*sqrt((Slip*Slip)+(tan(alpha)*tan(alpha)))))*(1-Slip))/...
    (2*sqrt(C_i*C_i*Slip*Slip+C_a*C_a*tan(alpha)*tan(alpha)));
if(S_f<1)
    f_S=S_f*(2-S_f);
else
    f_S=1;
end
F_SR_f=(C_a*tan(alpha)*f_S)/(1-Slip);
F_tR_f=(C_i*Slip*f_S)/(1-Slip);

%%Rear Tires
alpha=a_rR;

S_r=(mu*(Fz/3)*(1-(e_r*U_tr*sqrt((Slip*Slip)+(tan(alpha)*tan(alpha)))))*(1-Slip))/...
    (2*sqrt(C_i*C_i*Slip*Slip+C_a*C_a*tan(alpha)*tan(alpha)));
if(S_r<1)
    f_S=S_r*(2-S_r);
else
    f_S=1;
end
F_SR_r=(C_a*tan(alpha)*f_S)/(1-Slip);
F_tR_r=(C_i*Slip*f_S)/(1-Slip);

%%Middle Tires
alpha=a_mR;

S_m=(mu*(Fz/3)*(1-(e_r*U_tr*sqrt((Slip*Slip)+(tan(alpha)*tan(alpha)))))*(1-Slip))/...
    (2*sqrt(C_i*C_i*Slip*Slip+C_a*C_a*tan(alpha)*tan(alpha)));
if(S_m<1)
    f_S=S_m*(2-S_m);
else
    f_S=1;
end
F_SR_m=(C_a*tan(alpha)*f_S)/(1-Slip);
F_tR_m=(C_i*Slip*f_S)/(1-Slip);


F_SR=F_SR_f+F_SR_r+F_SR_m;
F_tR=F_tR_f+F_tR_r+F_tR_m;
F_R=[F_tR_f;F_tR_r;F_tR_m;F_SR_f;F_SR_r;F_SR_m];

== matlab function SS6_Estimation/Estimation Block/Fz_Calc_Esti ==
  data: U_dot input; V input; Fz_L output; Fz_R output; r input
function [Fz_L,Fz_R] = FzCalc(U_dot,V,r)
M=1280;Ms=1160;Izz=2500;Ixx=750;Ixz=0;a=1.203;b=1.217;hcg=0.5;e=0.2;Tw=1.33;R=0.3;I_t=2.1;
I_e=0.136;A_f=2.1;K_bf=0.55;zi1=13.56;z2=7.50;zi3=5.37;zi4=4.22;zi5=3.28;
Lbpsi=45000;Lbp=2600;C_a=20000;C_i=20000;mu=0.85;e_r=0.015;K_rsf=-0.05;K_rsr=0.1;
C1=-6.0;C2=59.16;C3=25;C_s1=1.38;K_rsf=0.444;C_d=0.32;d=0.014;n=0.85;
rho=1.204;g=9.81;


%NormalForceCalc
% Fz_f=(M*g/2)*((b/(a+b))-((U_dot-V*r)*hcg)/(g*(a+b)));
% Fz_r=(M*g/2)*((a/(a+b))+((U_dot-V*r)*hcg)/(g*(a+b)));
Fz_L=(M*g/2);
Fz_R=(M*g/2);

== matlab function SS6_Estimation/Estimation Block/VehicleEOMEsti ==
  data: U input; V input; U_dot output; V_dot output; r input; F_tL input; F_tR input; F_sL input; F_sR input; r_dot output; F_SL_f input; F_SL_r input; F_SL_m input; F_SR_f input; F_SR_r input; F_SR_m input
function [U_dot,V_dot,r_dot] = VehicleEOM(U,V,r,F_tL,F_tR,F_sL,F_sR,F_SL_f,F_SL_r,F_SL_m,F_SR_f,F_SR_r,F_SR_m)
M=1280;Ms=1160;Izz=2500;Ixx=750;Ixz=0;a=1.203;b=1.217;hcg=0.5;e=0.2;Tw=1.33;R=0.3;I_t=2.1;
I_e=0.136;A_f=2.1;K_bf=0.55;zi1=13.56;z2=7.50;zi3=5.37;zi4=4.22;zi5=3.28;
Lbpsi=45000;Lbp=2600;C_a=20000;C_i=20000;mu=0.85;e_r=0.015;K_rsf=-0.05;K_rsr=0.1;
C1=-6.0;C2=59.16;C3=25;C_s1=1.38;K_rsf=0.444;C_d=0.32;d=0.014;n=0.85;
rho=1.204;g=9.81;c=0.2;

F_t=(F_tL+F_tR);
%Vehicle Equations
% U_dot=(1/M)*((M*V*r)+F_t-(0.5*C_d*A_f*rho*U*U));
U_dot=(1/M)*((M*V*r)+F_t);

V_dot=(1/M)*((-M*U*r)+F_sL+F_sR);
% r_dot=(1/Izz)*(2*a*F_tL*sin(delta)+2*a*F_sL*cos(delta)-2*b*F_sR);
 r_dot=(1/(0.5*Izz))*(0.5*Tw*F_tL-0.5*Tw*F_tR+a*(F_SL_f+F_SR_f)-b*(F_SL_r+F_SR_r)-c*(F_SL_m+F_SR_m));
